simulink model "uut_vdif"  (R2012b)
settings: Solver=ode45  StartTime=0.0  StopTime=sim_time  RelTol=1e-3
libraries: xbsIndex_r4 x487, casper_library_delays x9, xps_library x1
(part 2 of 4)

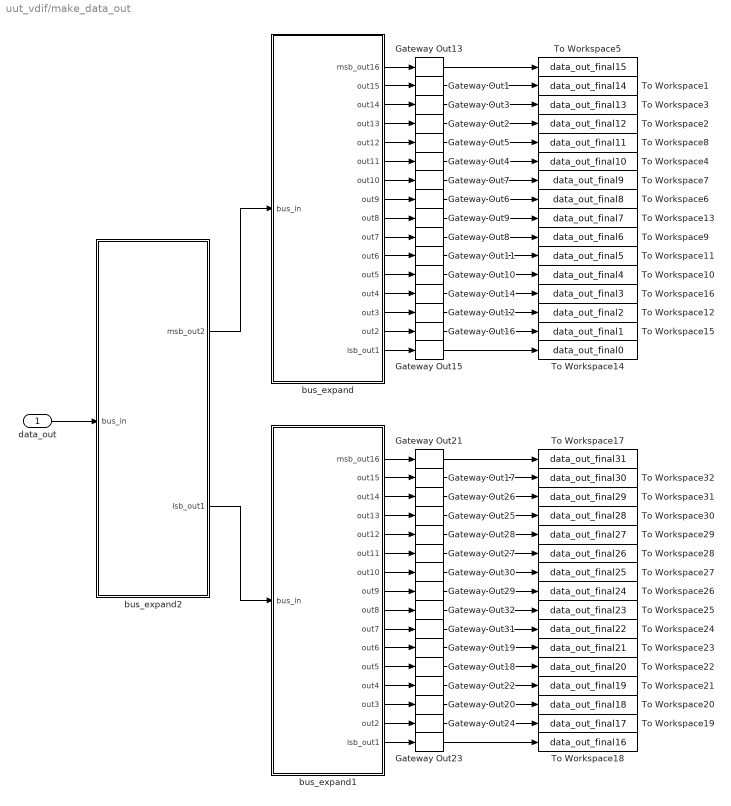
== system uut_vdif/make_data_out ==
  data_out : Inport
  Gateway Out{1..32} (32 alike) : xbsIndex_r4/Gateway Out  inherit_from_input=off  hdl_port=on  timing_constraint=None  locs_specified=off  LOCs={}  UseAsDAC=off  DACChannel='1'  block_type=gatewayout
  To Workspace1 : ToWorkspace  VariableName=data_out_final14  SampleTime=-1  SaveFormat=Timeseries
  To Workspace10 : ToWorkspace  VariableName=data_out_final4  SampleTime=-1  SaveFormat=Timeseries
  To Workspace11 : ToWorkspace  VariableName=data_out_final5  SampleTime=-1  SaveFormat=Timeseries
  To Workspace12 : ToWorkspace  VariableName=data_out_final2  SampleTime=-1  SaveFormat=Timeseries
  To Workspace13 : ToWorkspace  VariableName=data_out_final7  SampleTime=-1  SaveFormat=Timeseries
  To Workspace14 : ToWorkspace  VariableName=data_out_final0  SampleTime=-1  SaveFormat=Timeseries
  To Workspace15 : ToWorkspace  VariableName=data_out_final1  SampleTime=-1  SaveFormat=Timeseries
  To Workspace16 : ToWorkspace  VariableName=data_out_final3  SampleTime=-1  SaveFormat=Timeseries
  To Workspace17 : ToWorkspace  VariableName=data_out_final31  SampleTime=-1  SaveFormat=Timeseries
  To Workspace18 : ToWorkspace  VariableName=data_out_final16  SampleTime=-1  SaveFormat=Timeseries
  To Workspace19 : ToWorkspace  VariableName=data_out_final17  SampleTime=-1  SaveFormat=Timeseries
  To Workspace2 : ToWorkspace  VariableName=data_out_final12  SampleTime=-1  SaveFormat=Timeseries
  To Workspace20 : ToWorkspace  VariableName=data_out_final18  SampleTime=-1  SaveFormat=Timeseries
  To Workspace21 : ToWorkspace  VariableName=data_out_final19  SampleTime=-1  SaveFormat=Timeseries
  To Workspace22 : ToWorkspace  VariableName=data_out_final20  SampleTime=-1  SaveFormat=Timeseries
  To Workspace23 : ToWorkspace  VariableName=data_out_final21  SampleTime=-1  SaveFormat=Timeseries
  To Workspace24 : ToWorkspace  VariableName=data_out_final22  SampleTime=-1  SaveFormat=Timeseries
  To Workspace25 : ToWorkspace  VariableName=data_out_final23  SampleTime=-1  SaveFormat=Timeseries
  To Workspace26 : ToWorkspace  VariableName=data_out_final24  SampleTime=-1  SaveFormat=Timeseries
  To Workspace27 : ToWorkspace  VariableName=data_out_final25  SampleTime=-1  SaveFormat=Timeseries
  To Workspace28 : ToWorkspace  VariableName=data_out_final26  SampleTime=-1  SaveFormat=Timeseries
  To Workspace29 : ToWorkspace  VariableName=data_out_final27  SampleTime=-1  SaveFormat=Timeseries
  To Workspace3 : ToWorkspace  VariableName=data_out_final13  SampleTime=-1  SaveFormat=Timeseries
  To Workspace30 : ToWorkspace  VariableName=data_out_final28  SampleTime=-1  SaveFormat=Timeseries
  To Workspace31 : ToWorkspace  VariableName=data_out_final29  SampleTime=-1  SaveFormat=Timeseries
  To Workspace32 : ToWorkspace  VariableName=data_out_final30  SampleTime=-1  SaveFormat=Timeseries
  To Workspace4 : ToWorkspace  VariableName=data_out_final10  SampleTime=-1  SaveFormat=Timeseries
  To Workspace5 : ToWorkspace  VariableName=data_out_final15  SampleTime=-1  SaveFormat=Timeseries
  To Workspace6 : ToWorkspace  VariableName=data_out_final8  SampleTime=-1  SaveFormat=Timeseries
  To Workspace7 : ToWorkspace  VariableName=data_out_final9  SampleTime=-1  SaveFormat=Timeseries
  To Workspace8 : ToWorkspace  VariableName=data_out_final11  SampleTime=-1  SaveFormat=Timeseries
  To Workspace9 : ToWorkspace  VariableName=data_out_final6  SampleTime=-1  SaveFormat=Timeseries
  bus_expand : Subsystem  AncestorBlock=casper_library_flow_control/bus_expand  mask(bus_expand){mode=divisions of equal size, outputNum=16, outputWidth=2, outputBinaryPt=0, outputArithmeticType=0, show_format=off, outputToWorkspace=off, variablePrefix=out, outputToModelAsWell=on}
      mask prompts: outputNum "Number of outputs:"; outputWidth "Output width:"; outputBinaryPt "Output binary point position:"; outputArithmeticType "Output arithmetic type (ufix=0, fix=1, bool=2):"; show_format "Print format string?"; outputToWorkspace "Output to workspace?"; variablePrefix "Variable name prefix:"; outputToModelAsWell "Output to model as well?"
      mask help:
      | Expands a 'bus' made using a bus_create or Xilinx
      | concat block.
      | The input will be divided into the specified number
      | of outputs with the specified arithmetic types.
      | Divisions are made from most significant bit.
      mask init: same as uut_vdif/buffer_data/bus_expand
      settings: AttributesFormatString=16 outputs
      mask TypeOptions mode: divisions of equal size | divisions of arbitrary size
      mask Callback mode: bus_expand_callback();
      mask Callback outputWidth: bus_expand_callback();
      mask Callback outputToWorkspace: bus_expand_callback();
  bus_expand1 : Subsystem  AncestorBlock=casper_library_flow_control/bus_expand  mask(bus_expand){mode=divisions of equal size, outputNum=16, outputWidth=2, outputBinaryPt=0, outputArithmeticType=0, show_format=off, outputToWorkspace=off, variablePrefix=out, outputToModelAsWell=on}
      mask prompts: outputNum "Number of outputs:"; outputWidth "Output width:"; outputBinaryPt "Output binary point position:"; outputArithmeticType "Output arithmetic type (ufix=0, fix=1, bool=2):"; show_format "Print format string?"; outputToWorkspace "Output to workspace?"; variablePrefix "Variable name prefix:"; outputToModelAsWell "Output to model as well?"
      mask help:
      | Expands a 'bus' made using a bus_create or Xilinx
      | concat block.
      | The input will be divided into the specified number
      | of outputs with the specified arithmetic types.
      | Divisions are made from most significant bit.
      mask init: same as uut_vdif/buffer_data/bus_expand
      settings: AttributesFormatString=16 outputs
      mask TypeOptions mode: divisions of equal size | divisions of arbitrary size
      mask Callback mode: bus_expand_callback();
      mask Callback outputWidth: bus_expand_callback();
      mask Callback outputToWorkspace: bus_expand_callback();
  bus_expand2 : Subsystem  AncestorBlock=casper_library_flow_control/bus_expand  mask(bus_expand){mode=divisions of equal size, outputNum=2, outputWidth=32, outputBinaryPt=0, outputArithmeticType=0, show_format=off, outputToWorkspace=off, variablePrefix=out, outputToModelAsWell=on}
      mask prompts: outputNum "Number of outputs:"; outputWidth "Output width:"; outputBinaryPt "Output binary point position:"; outputArithmeticType "Output arithmetic type (ufix=0, fix=1, bool=2):"; show_format "Print format string?"; outputToWorkspace "Output to workspace?"; variablePrefix "Variable name prefix:"; outputToModelAsWell "Output to model as well?"
      mask help:
      | Expands a 'bus' made using a bus_create or Xilinx
      | concat block.
      | The input will be divided into the specified number
      | of outputs with the specified arithmetic types.
      | Divisions are made from most significant bit.
      mask init: same as uut_vdif/buffer_data/bus_expand
      settings: AttributesFormatString=2 outputs
      mask TypeOptions mode: divisions of equal size | divisions of arbitrary size
      mask Callback mode: bus_expand_callback();
      mask Callback outputWidth: bus_expand_callback();
      mask Callback outputToWorkspace: bus_expand_callback();
  wires:
  Gateway Out13/1 -> To Workspace5/1
  bus_expand/1(msb_out16) -> Gateway Out13/1
  bus_expand/2(out15) -> Gateway Out1/1
  Gateway Out1/1 -> To Workspace1/1
  Gateway Out3/1 -> To Workspace3/1
  bus_expand/3(out14) -> Gateway Out3/1
  bus_expand/4(out13) -> Gateway Out2/1
  Gateway Out2/1 -> To Workspace2/1
  Gateway Out5/1 -> To Workspace8/1
  bus_expand/5(out12) -> Gateway Out5/1
  bus_expand/6(out11) -> Gateway Out4/1
  Gateway Out4/1 -> To Workspace4/1
  Gateway Out7/1 -> To Workspace7/1
  bus_expand/7(out10) -> Gateway Out7/1
  bus_expand/8(out9) -> Gateway Out6/1
  Gateway Out6/1 -> To Workspace6/1
  Gateway Out9/1 -> To Workspace13/1
  bus_expand/9(out8) -> Gateway Out9/1
  bus_expand/10(out7) -> Gateway Out8/1
  Gateway Out8/1 -> To Workspace9/1
  Gateway Out11/1 -> To Workspace11/1
  bus_expand/11(out6) -> Gateway Out11/1
  bus_expand/12(out5) -> Gateway Out10/1
  Gateway Out10/1 -> To Workspace10/1
  Gateway Out14/1 -> To Workspace16/1
  bus_expand/13(out4) -> Gateway Out14/1
  bus_expand/14(out3) -> Gateway Out12/1
  Gateway Out12/1 -> To Workspace12/1
  Gateway Out16/1 -> To Workspace15/1
  bus_expand/15(out2) -> Gateway Out16/1
  bus_expand/16(lsb_out1) -> Gateway Out15/1
  Gateway Out15/1 -> To Workspace14/1
  bus_expand1/1(msb_out16) -> Gateway Out21/1
  bus_expand1/2(out15) -> Gateway Out17/1
  bus_expand1/3(out14) -> Gateway Out26/1
  bus_expand1/4(out13) -> Gateway Out25/1
  bus_expand1/5(out12) -> Gateway Out28/1
  bus_expand1/6(out11) -> Gateway Out27/1
  bus_expand1/7(out10) -> Gateway Out30/1
  bus_expand1/8(out9) -> Gateway Out29/1
  bus_expand1/9(out8) -> Gateway Out32/1
  bus_expand1/10(out7) -> Gateway Out31/1
  bus_expand1/11(out6) -> Gateway Out19/1
  bus_expand1/12(out5) -> Gateway Out18/1
  bus_expand1/13(out4) -> Gateway Out22/1
  bus_expand1/14(out3) -> Gateway Out20/1
  bus_expand1/15(out2) -> Gateway Out24/1
  bus_expand1/16(lsb_out1) -> Gateway Out23/1
  data_out/1 -> bus_expand2/1(bus_in)
  bus_expand2/1(msb_out2) -> bus_expand/1(bus_in)
  bus_expand2/2(lsb_out1) -> bus_expand1/1(bus_in)
  Gateway Out21/1 -> To Workspace17/1
  Gateway Out17/1 -> To Workspace32/1
  Gateway Out26/1 -> To Workspace31/1
  Gateway Out25/1 -> To Workspace30/1
  Gateway Out28/1 -> To Workspace29/1
  Gateway Out27/1 -> To Workspace28/1
  Gateway Out30/1 -> To Workspace27/1
  Gateway Out29/1 -> To Workspace26/1
  Gateway Out32/1 -> To Workspace25/1
  Gateway Out31/1 -> To Workspace24/1
  Gateway Out19/1 -> To Workspace23/1
  Gateway Out18/1 -> To Workspace22/1
  Gateway Out22/1 -> To Workspace21/1
  Gateway Out20/1 -> To Workspace20/1
  Gateway Out24/1 -> To Workspace19/1
  Gateway Out23/1 -> To Workspace18/1

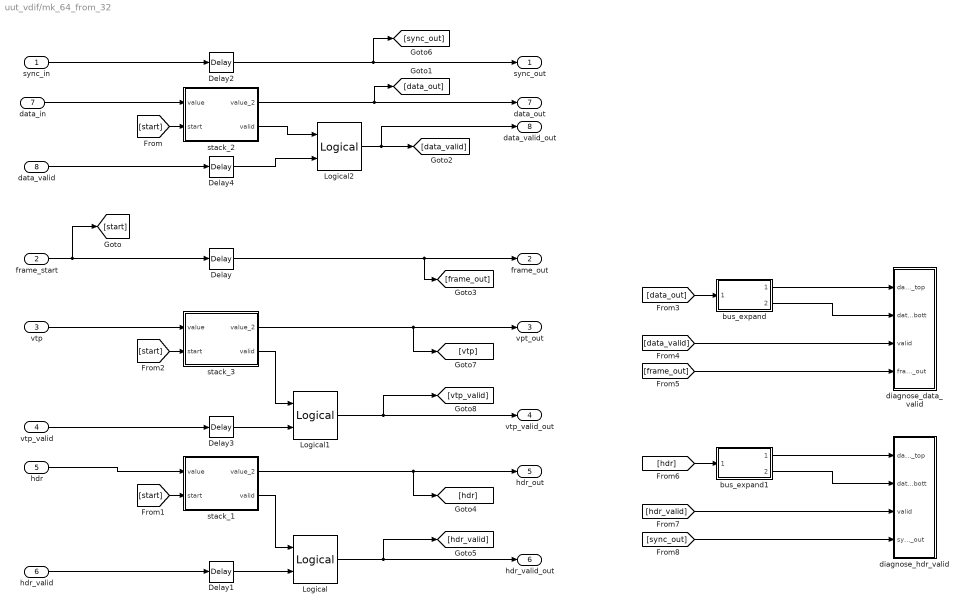
== system uut_vdif/mk_64_from_32 ==
  sync_in : Inport
  frame_start : Inport  Port=2
  vtp : Inport  Port=3
  vtp_valid : Inport  Port=4
  hdr : Inport  Port=5
  hdr_valid : Inport  Port=6
  data_in : Inport  Port=7
  data_valid : Inport  Port=8
  Delay{,1..4} (5 alike) : xbsIndex_r4/Delay  rst=off  infoeditControl=Selection of Reset will increase slice count due to use of real FFs and instead of SRLs  en=off  latency=2  dbl_ovrd=off  reg_retiming=off  block_type=delay
  Logical : xbsIndex_r4/Logical  logical_function=AND  inputs=2  en=off  latency=0  precision=Full  arith_type=Unsigned  n_bits=16  bin_pt=0  align_bp=on  dbl_ovrd=off  block_type=logical
  Logical1 : xbsIndex_r4/Logical  logical_function=AND  inputs=2  en=off  latency=0  precision=Full  arith_type=Unsigned  n_bits=16  bin_pt=0  align_bp=on  dbl_ovrd=off  block_type=logical
  Logical2 : xbsIndex_r4/Logical  logical_function=AND  inputs=2  en=off  latency=0  precision=Full  arith_type=Unsigned  n_bits=16  bin_pt=0  align_bp=on  dbl_ovrd=off  block_type=logical
  bus_expand : Subsystem  AncestorBlock=casper_library_flow_control/bus_expand  mask(bus_expand){mode=divisions of equal size, outputNum=2, outputWidth=32, outputBinaryPt=0, outputArithmeticType=0, show_format=off, outputToWorkspace=off, variablePrefix=out, outputToModelAsWell=on}
      mask prompts: outputNum "Number of outputs:"; outputWidth "Output width:"; outputBinaryPt "Output binary point position:"; outputArithmeticType "Output arithmetic type (ufix=0, fix=1, bool=2):"; show_format "Print format string?"; outputToWorkspace "Output to workspace?"; variablePrefix "Variable name prefix:"; outputToModelAsWell "Output to model as well?"
      mask help:
      | Expands a 'bus' made using a bus_create or Xilinx
      | concat block.
      | The input will be divided into the specified number
      | of outputs with the specified arithmetic types.
      | Divisions are made from most significant bit.
      mask init: same as uut_vdif/buffer_data/bus_expand
      settings: AttributesFormatString=2 outputs
      mask TypeOptions mode: divisions of equal size | divisions of arbitrary size
      mask Callback mode: bus_expand_callback();
      mask Callback outputWidth: bus_expand_callback();
      mask Callback outputToWorkspace: bus_expand_callback();
  bus_expand1 : Subsystem  AncestorBlock=casper_library_flow_control/bus_expand  mask(bus_expand){mode=divisions of equal size, outputNum=2, outputWidth=32, outputBinaryPt=0, outputArithmeticType=0, show_format=off, outputToWorkspace=off, variablePrefix=out, outputToModelAsWell=on}
      mask prompts: outputNum "Number of outputs:"; outputWidth "Output width:"; outputBinaryPt "Output binary point position:"; outputArithmeticType "Output arithmetic type (ufix=0, fix=1, bool=2):"; show_format "Print format string?"; outputToWorkspace "Output to workspace?"; variablePrefix "Variable name prefix:"; outputToModelAsWell "Output to model as well?"
      mask help:
      | Expands a 'bus' made using a bus_create or Xilinx
      | concat block.
      | The input will be divided into the specified number
      | of outputs with the specified arithmetic types.
      | Divisions are made from most significant bit.
      mask init: same as uut_vdif/buffer_data/bus_expand
      settings: AttributesFormatString=2 outputs
      mask TypeOptions mode: divisions of equal size | divisions of arbitrary size
      mask Callback mode: bus_expand_callback();
      mask Callback outputWidth: bus_expand_callback();
      mask Callback outputToWorkspace: bus_expand_callback();
  diagnose_data_valid : Subsystem
  diagnose_hdr_valid : Subsystem
  stack_1 : Subsystem
      mask help: stacks 2 samples together, based on a flag that indicates the start or the first sample of data to be stacked. outputs the stacked data and a valid signal, such that on any given valid signal the data represents the newest data in the top half and the oldest data in the lower half. Therefore given a data stream starting with 0, increasing by 1 every clock cycle I would expect the first data valid to indicate a piece of data with the value 0 in the low bits, 1 in the high, and the next sample having 2 in the low bits 3 in the high, etc.
  stack_2 : Subsystem
      mask help: stacks 2 samples together, based on a flag that indicates the start or the first sample of data to be stacked. outputs the stacked data and a valid signal, such that on any given valid signal the data represents the newest data in the top half and the oldest data in the lower half. Therefore given a data stream starting with 0, increasing by 1 every clock cycle I would expect the first data valid to indicate a piece of data with the value 0 in the low bits, 1 in the high, and the next sample having 2 in the low bits 3 in the high, etc.
  stack_3 : Subsystem
      mask help: stacks 2 samples together, based on a flag that indicates the start or the first sample of data to be stacked. outputs the stacked data and a valid signal, such that on any given valid signal the data represents the newest data in the top half and the oldest data in the lower half. Therefore given a data stream starting with 0, increasing by 1 every clock cycle I would expect the first data valid to indicate a piece of data with the value 0 in the low bits, 1 in the high, and the next sample having 2 in the low bits 3 in the high, etc.
  sync_out : Outport
  frame_out : Outport  Port=2
  vpt_out : Outport  Port=3
  vtp_valid_out : Outport  Port=4
  hdr_out : Outport  Port=5
  hdr_valid_out : Outport  Port=6
  data_out : Outport  Port=7
  data_valid_out : Outport  Port=8
  wires:
  data_in/1 -> stack_2/1(value)
  frame_start/1 -> [start], Delay/1
  [start] -> stack_2/2(start)
  sync_in/1 -> Delay2/1
  stack_2/1(value_2) -> data_out/1, [data_out]
  [start] -> stack_1/2(start)
  stack_1/1(value_2) -> hdr_out/1, [hdr]
  stack_1/2(valid) -> Logical/1
  Delay/1 -> [frame_out], frame_out/1
  bus_expand/2(lsb_out1) -> diagnose_data_valid/2(data_bott)
  bus_expand/1(msb_out2) -> diagnose_data_valid/1(data_top)
  [data_valid] -> diagnose_data_valid/3(valid)
  [frame_out] -> diagnose_data_valid/4(frame_start_out)
  [data_out] -> bus_expand/1(bus_in)
  bus_expand1/2(lsb_out1) -> diagnose_hdr_valid/2(data_bott)
  bus_expand1/1(msb_out2) -> diagnose_hdr_valid/1(data_top)
  [hdr_valid] -> diagnose_hdr_valid/3(valid)
  [sync_out] -> diagnose_hdr_valid/4(sync_out)
  [hdr] -> bus_expand1/1(bus_in)
  Logical/1 -> hdr_valid_out/1, [hdr_valid]
  Delay1/1 -> Logical/2
  Delay2/1 -> [sync_out], sync_out/1
  [start] -> stack_3/2(start)
  stack_3/1(value_2) -> vpt_out/1, [vtp]
  stack_3/2(valid) -> Logical1/1
  Logical1/1 -> vtp_valid_out/1, [vtp_valid]
  Delay3/1 -> Logical1/2
  vtp/1 -> stack_3/1(value)
  vtp_valid/1 -> Delay3/1
  hdr/1 -> stack_1/1(value)
  hdr_valid/1 -> Delay1/1
  data_valid/1 -> Delay4/1
  Delay4/1 -> Logical2/2
  stack_2/2(valid) -> Logical2/1
  Logical2/1 -> data_valid_out/1, [data_valid]

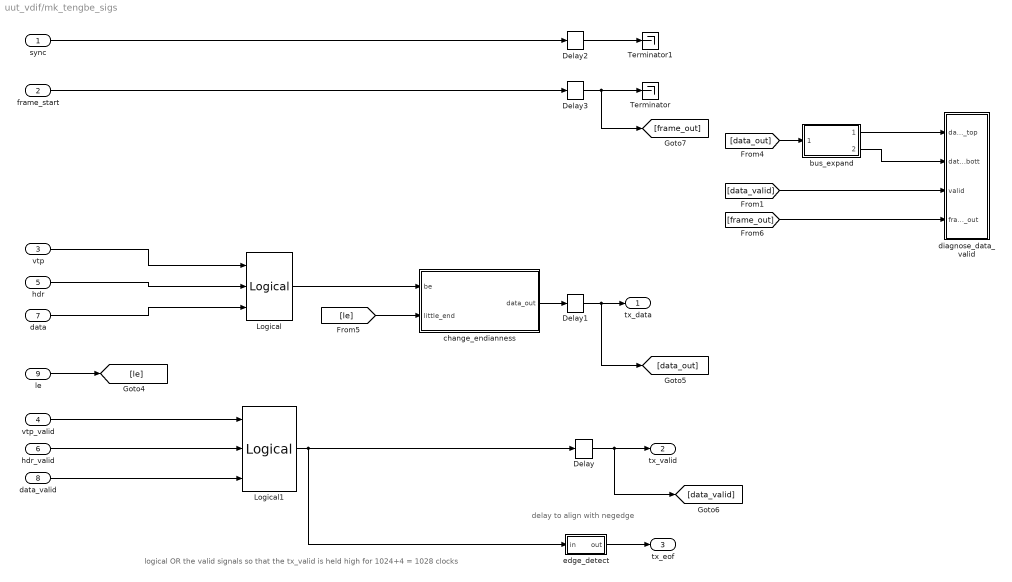
== system uut_vdif/mk_tengbe_sigs ==
  note: logical OR the valid signals so that the
      | tx_valid is held high for 1024+4 = 1028 clocks
  note: delay to align with
      | negedge
  sync : Inport
  frame_start : Inport  Port=2
  vtp : Inport  Port=3
  vtp_valid : Inport  Port=4
  hdr : Inport  Port=5
  hdr_valid : Inport  Port=6
  data : Inport  Port=7
  data_valid : Inport  Port=8
  le : Inport  Port=9
  Delay{,1..3} (4 alike) : xbsIndex_r4/Delay  rst=off  infoeditControl=Selection of Reset will increase slice count due to use of real FFs and instead of SRLs  en=off  latency=1  dbl_ovrd=off  reg_retiming=off  block_type=delay
  Logical : xbsIndex_r4/Logical  logical_function=XOR  inputs=3  en=off  latency=0  precision=Full  arith_type=Unsigned  n_bits=16  bin_pt=0  align_bp=on  dbl_ovrd=off  block_type=logical
  Logical1 : xbsIndex_r4/Logical  logical_function=XOR  inputs=3  en=off  latency=0  precision=Full  arith_type=Unsigned  n_bits=16  bin_pt=0  align_bp=on  dbl_ovrd=off  block_type=logical
  Terminator : Terminator
  Terminator1 : Terminator
  bus_expand : Subsystem  AncestorBlock=casper_library_flow_control/bus_expand  mask(bus_expand){mode=divisions of equal size, outputNum=2, outputWidth=32, outputBinaryPt=0, outputArithmeticType=0, show_format=off, outputToWorkspace=off, variablePrefix=out, outputToModelAsWell=on}
      mask prompts: outputNum "Number of outputs:"; outputWidth "Output width:"; outputBinaryPt "Output binary point position:"; outputArithmeticType "Output arithmetic type (ufix=0, fix=1, bool=2):"; show_format "Print format string?"; outputToWorkspace "Output to workspace?"; variablePrefix "Variable name prefix:"; outputToModelAsWell "Output to model as well?"
      mask help:
      | Expands a 'bus' made using a bus_create or Xilinx
      | concat block.
      | The input will be divided into the specified number
      | of outputs with the specified arithmetic types.
      | Divisions are made from most significant bit.
      mask init: same as uut_vdif/buffer_data/bus_expand
      settings: AttributesFormatString=2 outputs
      mask TypeOptions mode: divisions of equal size | divisions of arbitrary size
      mask Callback mode: bus_expand_callback();
      mask Callback outputWidth: bus_expand_callback();
      mask Callback outputToWorkspace: bus_expand_callback();
  change_endianness : Subsystem
  diagnose_data_valid : Subsystem
  edge_detect : Subsystem  AncestorBlock=casper_library_misc/edge_detect  mask(edge_detect){edge=Falling, polarity=Active High, x_in=[0 0.08 0.08 0.16 0.16 0.24 0.24 0.32 0.32 0.4], y_in=[-1 -1  1  1  1  1  1  1  1  1], x_out=[0.6 0.68 0.68 0.76 0.76 0.84 0.84 0.92 0.92 1], y_out=[-1 -1  1  1 -1 -1 -1 -1 -1 -1]}
      mask prompts: edge "Edge Type"; polarity "Output Polarity"; x_in "Input X Positions"; y_in "Input Y Positions"; x_out "Output X Positions"; y_out "Output Y Positions"
      mask help: Output is active for one-cycle after each edge of the specified type (i.e. rising, falling or both).
      mask init:
      | edge_detect_init(gcb,...
      |     'edge',edge,...
      |     'polarity',polarity,...
      |     'x_in',x_in,...
      |     'x_out',x_out,...
      |     'y_in',y_in,...
      |     'y_out',y_out);
      | 
      | x_in_num=str2num(getfield(getfield(get_param(gcb,'UserData'),'parameters'),'x_in'));
      | x_out_num=str2num(getfield(getfield(get_param(gcb,'UserData'),'parameters'),'x_out'));
      | y_in_num=str2num(getfield(getfield(get_param(gcb,'UserData'),'parameters'),'y_in'));
      | y_out_num=str2num(getfield(getfield(get_param(gcb,'UserData'),'parameters'),'y_out'));
      settings: AttributesFormatString=|
      | falling edges
      | active high
      mask Help: Output is active for one-cycle after each edge of the specified type (i.e. rising, falling, or both).  Latency is zero.
      mask TypeOptions edge: Rising | Falling | Both
      mask TypeOptions polarity: Active High | Active Low
      mask Display:
      | plot(x_in_num,0.5+y_in_num*0.2);
      | plot(x_out_num,0.5+y_out_num*0.2);
  tx_data : Outport
  tx_valid : Outport  Port=2
  tx_eof : Outport  Port=3
  wires:
  edge_detect/1(out) -> tx_eof/1
  Logical1/1 -> edge_detect/1(in), Delay/1
  Delay/1 -> [data_valid], tx_valid/1
  Logical/1 -> change_endianness/1(be)
  change_endianness/1(data_out) -> Delay1/1
  [le] -> change_endianness/2(little_end)
  Delay2/1 -> Terminator1/1
  sync/1 -> Delay2/1
  Delay1/1 -> [data_out], tx_data/1
  frame_start/1 -> Delay3/1
  Delay3/1 -> [frame_out], Terminator/1
  bus_expand/2(lsb_out1) -> diagnose_data_valid/2(data_bott)
  bus_expand/1(msb_out2) -> diagnose_data_valid/1(data_top)
  [data_valid] -> diagnose_data_valid/3(valid)
  [frame_out] -> diagnose_data_valid/4(frame_start_out)
  [data_out] -> bus_expand/1(bus_in)
  hdr/1 -> Logical/2
  vtp/1 -> Logical/1
  data/1 -> Logical/3
  le/1 -> [le]
  vtp_valid/1 -> Logical1/1
  hdr_valid/1 -> Logical1/2
  data_valid/1 -> Logical1/3

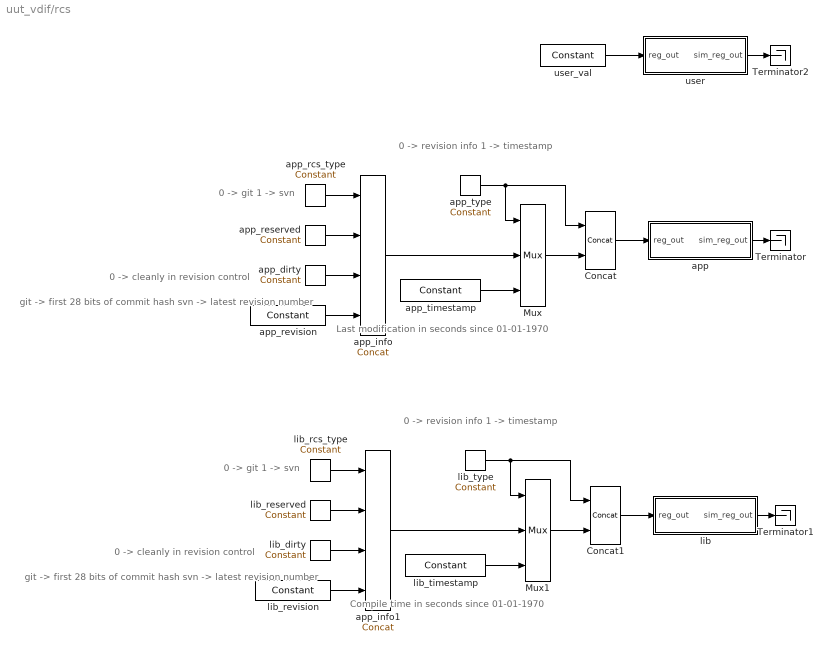
== system uut_vdif/rcs ==
  note: 0 -> revision info
      | 1 -> timestamp
  note: Last modification
      | in seconds since
      | 01-01-1970
  note: 0 -> git
      | 1 -> svn
  note: 0 -> cleanly in revision control
  note: git -> first 28 bits of commit hash
      | svn -> latest revision number
  note: 0 -> revision info
      | 1 -> timestamp
  note: Compile time
      | in seconds since
      | 01-01-1970
  note: 0 -> git
      | 1 -> svn
  note: 0 -> cleanly in revision control
  note: git -> first 28 bits of commit hash
      | svn -> latest revision number
  Concat : xbsIndex_r4/Concat  num_inputs=2  dbl_ovrd=off  block_type=concat
  Concat1 : xbsIndex_r4/Concat  num_inputs=2  dbl_ovrd=off  block_type=concat
  Mux : xbsIndex_r4/Mux  inputs=2  en=off  latency=0  precision=Full  arith_type=Unsigned  n_bits=16  bin_pt=14  quantization=Truncate  overflow=Wrap  dbl_ovrd=off  block_type=mux
      settings: block_version=11.4
  Mux1 : xbsIndex_r4/Mux  inputs=2  en=off  latency=0  precision=Full  arith_type=Unsigned  n_bits=16  bin_pt=14  quantization=Truncate  overflow=Wrap  dbl_ovrd=off  block_type=mux
      settings: block_version=11.4
  Terminator : Terminator
  Terminator1 : Terminator
  Terminator2 : Terminator
  app : Subsystem  Tag=xps:sw_reg  mask{io_dir=To Processor, arith_type=Unsigned, bitwidth=32, bin_pt=0, sample_period=1, latency=0}
      mask prompts: io_dir "I/O direction"; arith_type "Data Type"; bitwidth "Data bitwidth"; bin_pt "Data binary point"; sample_period "Sample period"
      mask init:
      | gw_name = clear_name(gcb);
      | config.source = str2func('software_register_init');
      | config.toplevel = gcb;
      | xBlock( config, {io_dir, arith_type, bitwidth, bin_pt, ... 
      |     sample_period, gw_name, latency});
      mask TypeOptions io_dir: From Processor | To Processor
      mask TypeOptions arith_type: Unsigned | Signed  (2's comp)
  app_dirty : xbsIndex_r4/Constant  const=1  gui_display_data_type=Fixed-point  arith_type=Unsigned  n_bits=1  bin_pt=0  preci_type=Single  exp_width=8  frac_width=24  explicit_period=on  period=1  equ=P=C  opselect=C  inp2=PCIN>>17  opr=+  inp1=P  carry=CIN  dbl_ovrd=off  block_type=constant
      settings: block_version=11.4
  app_info : xbsIndex_r4/Concat  num_inputs=4  dbl_ovrd=off  block_type=concat
  app_info1 : xbsIndex_r4/Concat  num_inputs=4  dbl_ovrd=off  block_type=concat
  app_rcs_type : xbsIndex_r4/Constant  const=0  gui_display_data_type=Fixed-point  arith_type=Unsigned  n_bits=1  bin_pt=0  preci_type=Single  exp_width=8  frac_width=24  explicit_period=on  period=1  equ=P=C  opselect=C  inp2=PCIN>>17  opr=+  inp1=P  carry=CIN  dbl_ovrd=off  block_type=constant
      settings: block_version=11.4
  app_reserved : xbsIndex_r4/Constant  const=0  gui_display_data_type=Fixed-point  arith_type=Unsigned  n_bits=1  bin_pt=0  preci_type=Single  exp_width=8  frac_width=24  explicit_period=on  period=1  equ=P=C  opselect=C  inp2=PCIN>>17  opr=+  inp1=P  carry=CIN  dbl_ovrd=off  block_type=constant
      settings: block_version=11.4
  app_revision : xbsIndex_r4/Constant  const=0  gui_display_data_type=Fixed-point  arith_type=Unsigned  n_bits=28  bin_pt=0  preci_type=Single  exp_width=8  frac_width=24  explicit_period=on  period=1  equ=P=C  opselect=C  inp2=PCIN>>17  opr=+  inp1=P  carry=CIN  dbl_ovrd=off  block_type=constant
      settings: block_version=11.4
  app_timestamp : xbsIndex_r4/Constant  const=1440776925  gui_display_data_type=Fixed-point  arith_type=Unsigned  n_bits=31  bin_pt=0  preci_type=Single  exp_width=8  frac_width=24  explicit_period=on  period=1  equ=P=C  opselect=C  inp2=PCIN>>17  opr=+  inp1=P  carry=CIN  dbl_ovrd=off  block_type=constant
      settings: block_version=11.4
  app_type : xbsIndex_r4/Constant  const=1  gui_display_data_type=Fixed-point  arith_type=Unsigned  n_bits=1  bin_pt=0  preci_type=Single  exp_width=8  frac_width=24  explicit_period=on  period=1  equ=P=C  opselect=C  inp2=PCIN>>17  opr=+  inp1=P  carry=CIN  dbl_ovrd=off  block_type=constant
      settings: block_version=11.4
  lib : Subsystem  Tag=xps:sw_reg  mask{io_dir=To Processor, arith_type=Unsigned, bitwidth=32, bin_pt=0, sample_period=1, latency=0}
      mask prompts: io_dir "I/O direction"; arith_type "Data Type"; bitwidth "Data bitwidth"; bin_pt "Data binary point"; sample_period "Sample period"
      mask init:
      | gw_name = clear_name(gcb);
      | config.source = str2func('software_register_init');
      | config.toplevel = gcb;
      | xBlock( config, {io_dir, arith_type, bitwidth, bin_pt, ... 
      |     sample_period, gw_name, latency});
      mask TypeOptions io_dir: From Processor | To Processor
      mask TypeOptions arith_type: Unsigned | Signed  (2's comp)
  lib_dirty : xbsIndex_r4/Constant  const=1  gui_display_data_type=Fixed-point  arith_type=Unsigned  n_bits=1  bin_pt=0  preci_type=Single  exp_width=8  frac_width=24  explicit_period=on  period=1  equ=P=C  opselect=C  inp2=PCIN>>17  opr=+  inp1=P  carry=CIN  dbl_ovrd=off  block_type=constant
      settings: block_version=11.4
  lib_rcs_type : xbsIndex_r4/Constant  const=0  gui_display_data_type=Fixed-point  arith_type=Unsigned  n_bits=1  bin_pt=0  preci_type=Single  exp_width=8  frac_width=24  explicit_period=on  period=1  equ=P=C  opselect=C  inp2=PCIN>>17  opr=+  inp1=P  carry=CIN  dbl_ovrd=off  block_type=constant
      settings: block_version=11.4
  lib_reserved : xbsIndex_r4/Constant  const=0  gui_display_data_type=Fixed-point  arith_type=Unsigned  n_bits=1  bin_pt=0  preci_type=Single  exp_width=8  frac_width=24  explicit_period=on  period=1  equ=P=C  opselect=C  inp2=PCIN>>17  opr=+  inp1=P  carry=CIN  dbl_ovrd=off  block_type=constant
      settings: block_version=11.4
  lib_revision : xbsIndex_r4/Constant  const=hex2dec('a288ff3')  gui_display_data_type=Fixed-point  arith_type=Unsigned  n_bits=28  bin_pt=0  preci_type=Single  exp_width=8  frac_width=24  explicit_period=on  period=1  equ=P=C  opselect=C  inp2=PCIN>>17  opr=+  inp1=P  carry=CIN  dbl_ovrd=off  block_type=constant
      settings: block_version=11.4
  lib_timestamp : xbsIndex_r4/Constant  const=1440763282  gui_display_data_type=Fixed-point  arith_type=Unsigned  n_bits=31  bin_pt=0  preci_type=Single  exp_width=8  frac_width=24  explicit_period=on  period=1  equ=P=C  opselect=C  inp2=PCIN>>17  opr=+  inp1=P  carry=CIN  dbl_ovrd=off  block_type=constant
      settings: block_version=11.4
  lib_type : xbsIndex_r4/Constant  const=0  gui_display_data_type=Fixed-point  arith_type=Unsigned  n_bits=1  bin_pt=0  preci_type=Single  exp_width=8  frac_width=24  explicit_period=on  period=1  equ=P=C  opselect=C  inp2=PCIN>>17  opr=+  inp1=P  carry=CIN  dbl_ovrd=off  block_type=constant
      settings: block_version=11.4
  user : Subsystem  Tag=xps:sw_reg  mask{io_dir=To Processor, arith_type=Unsigned, bitwidth=32, bin_pt=0, sample_period=1, latency=0}
      mask prompts: io_dir "I/O direction"; arith_type "Data Type"; bitwidth "Data bitwidth"; bin_pt "Data binary point"; sample_period "Sample period"
      mask init:
      | gw_name = clear_name(gcb);
      | config.source = str2func('software_register_init');
      | config.toplevel = gcb;
      | xBlock( config, {io_dir, arith_type, bitwidth, bin_pt, ... 
      |     sample_period, gw_name, latency});
      mask TypeOptions io_dir: From Processor | To Processor
      mask TypeOptions arith_type: Unsigned | Signed  (2's comp)
  user_val : xbsIndex_r4/Constant  const=user_val  gui_display_data_type=Fixed-point  arith_type=Unsigned  n_bits=32  bin_pt=0  preci_type=Single  exp_width=8  frac_width=24  explicit_period=off  period=1  equ=P=C  opselect=C  inp2=PCIN>>17  opr=+  inp1=P  carry=CIN  dbl_ovrd=off  block_type=constant
      settings: block_version=11.4
  wires:
  app/1(sim_reg_out) -> Terminator/1
  user/1(sim_reg_out) -> Terminator2/1
  user_val/1 -> user/1(reg_out)
  app_rcs_type/1 -> app_info/1
  app_reserved/1 -> app_info/2
  app_dirty/1 -> app_info/3
  app_revision/1 -> app_info/4
  app_type/1 -> Concat/1, Mux/1
  app_info/1 -> Mux/2
  app_timestamp/1 -> Mux/3
  Mux/1 -> Concat/2
  Concat/1 -> app/1(reg_out)
  lib/1(sim_reg_out) -> Terminator1/1
  lib_rcs_type/1 -> app_info1/1
  lib_reserved/1 -> app_info1/2
  lib_dirty/1 -> app_info1/3
  lib_revision/1 -> app_info1/4
  lib_type/1 -> Concat1/1, Mux1/1
  app_info1/1 -> Mux1/2
  lib_timestamp/1 -> Mux1/3
  Mux1/1 -> Concat1/2
  Concat1/1 -> lib/1(reg_out)

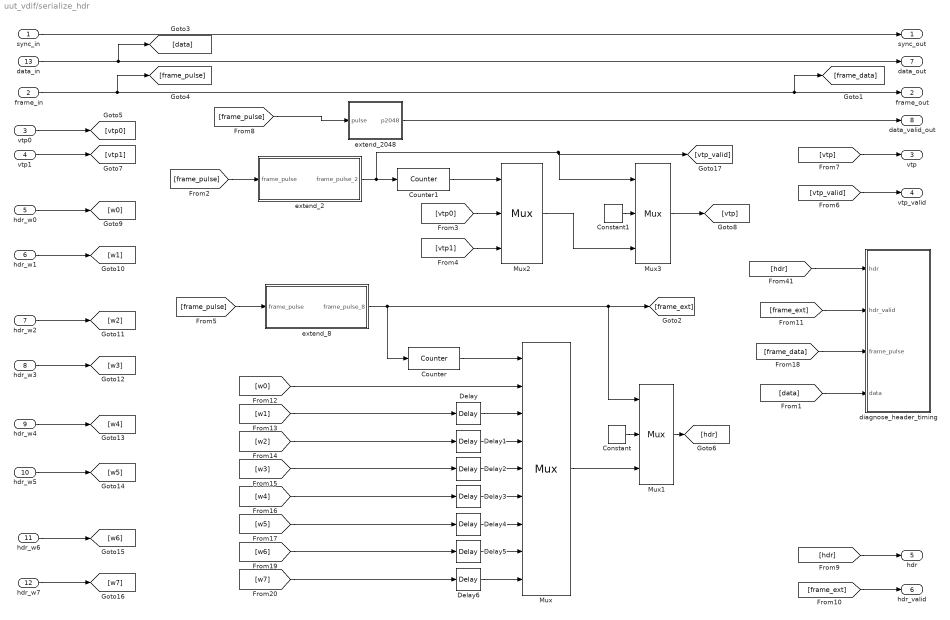
== system uut_vdif/serialize_hdr ==
  sync_in : Inport
  frame_in : Inport  Port=2
  vtp0 : Inport  Port=3
  vtp1 : Inport  Port=4
  " hdr_w0" : Inport  Port=5
  " hdr_w1" : Inport  Port=6
  " hdr_w2" : Inport  Port=7
  " hdr_w3" : Inport  Port=8
  " hdr_w4" : Inport  Port=9
  " hdr_w5" : Inport  Port=10
  " hdr_w6" : Inport  Port=11
  " hdr_w7" : Inport  Port=12
  " data_in" : Inport  Port=13
  Constant : xbsIndex_r4/Constant  const=0  gui_display_data_type=Fixed-point  arith_type=Unsigned  n_bits=32  bin_pt=0  preci_type=Single  exp_width=8  frac_width=24  explicit_period=on  period=1  equ=P=C  opselect=C  inp2=PCIN>>17  opr=+  inp1=P  carry=CIN  dbl_ovrd=off  block_type=constant
  Constant1 : xbsIndex_r4/Constant  const=0  gui_display_data_type=Fixed-point  arith_type=Unsigned  n_bits=32  bin_pt=0  preci_type=Single  exp_width=8  frac_width=24  explicit_period=on  period=1  equ=P=C  opselect=C  inp2=PCIN>>17  opr=+  inp1=P  carry=CIN  dbl_ovrd=off  block_type=constant
  Counter : xbsIndex_r4/Counter  cnt_type=Free Running  cnt_to=Inf  operation=Up  start_count=0  cnt_by_val=1  arith_type=Unsigned  n_bits=3  bin_pt=0  load_pin=off  rst=off  en=on  explicit_period=on  period=1  dbl_ovrd=off  use_behavioral_HDL=off  implementation=Fabric  block_type=counter
  Counter1 : xbsIndex_r4/Counter  cnt_type=Free Running  cnt_to=Inf  operation=Up  start_count=0  cnt_by_val=1  arith_type=Unsigned  n_bits=1  bin_pt=0  load_pin=off  rst=off  en=on  explicit_period=on  period=1  dbl_ovrd=off  use_behavioral_HDL=off  implementation=Fabric  block_type=counter
  Delay : xbsIndex_r4/Delay  rst=off  infoeditControl=Selection of Reset will increase slice count due to use of real FFs and instead of SRLs  en=off  latency=1  dbl_ovrd=off  reg_retiming=off  block_type=delay
  Delay1 : xbsIndex_r4/Delay  rst=off  infoeditControl=Selection of Reset will increase slice count due to use of real FFs and instead of SRLs  en=off  latency=2  dbl_ovrd=off  reg_retiming=off  block_type=delay
  Delay2 : xbsIndex_r4/Delay  rst=off  infoeditControl=Selection of Reset will increase slice count due to use of real FFs and instead of SRLs  en=off  latency=3  dbl_ovrd=off  reg_retiming=off  block_type=delay
  Delay3 : xbsIndex_r4/Delay  rst=off  infoeditControl=Selection of Reset will increase slice count due to use of real FFs and instead of SRLs  en=off  latency=4  dbl_ovrd=off  reg_retiming=off  block_type=delay
  Delay4 : xbsIndex_r4/Delay  rst=off  infoeditControl=Selection of Reset will increase slice count due to use of real FFs and instead of SRLs  en=off  latency=5  dbl_ovrd=off  reg_retiming=off  block_type=delay
  Delay5 : xbsIndex_r4/Delay  rst=off  infoeditControl=Selection of Reset will increase slice count due to use of real FFs and instead of SRLs  en=off  latency=6  dbl_ovrd=off  reg_retiming=off  block_type=delay
  Delay6 : xbsIndex_r4/Delay  rst=off  infoeditControl=Selection of Reset will increase slice count due to use of real FFs and instead of SRLs  en=off  latency=7  dbl_ovrd=off  reg_retiming=off  block_type=delay
  Mux : xbsIndex_r4/Mux  inputs=8  en=off  latency=0  precision=Full  arith_type=Unsigned  n_bits=16  bin_pt=14  quantization=Truncate  overflow=Wrap  dbl_ovrd=off  block_type=mux
  Mux1 : xbsIndex_r4/Mux  inputs=2  en=off  latency=0  precision=Full  arith_type=Unsigned  n_bits=16  bin_pt=14  quantization=Truncate  overflow=Wrap  dbl_ovrd=off  block_type=mux
  Mux2 : xbsIndex_r4/Mux  inputs=2  en=off  latency=0  precision=Full  arith_type=Unsigned  n_bits=16  bin_pt=14  quantization=Truncate  overflow=Wrap  dbl_ovrd=off  block_type=mux
  Mux3 : xbsIndex_r4/Mux  inputs=2  en=off  latency=0  precision=Full  arith_type=Unsigned  n_bits=16  bin_pt=14  quantization=Truncate  overflow=Wrap  dbl_ovrd=off  block_type=mux
  diagnose_header_timing : Subsystem
  extend_2 : Subsystem
  extend_2048 : Subsystem
  extend_8 : Subsystem
  sync_out : Outport
  frame_out : Outport  Port=2
  vtp : Outport  Port=3
  vtp_valid : Outport  Port=4
  hdr : Outport  Port=5
  hdr_valid : Outport  Port=6
  data_out : Outport  Port=7
  data_valid_out : Outport  Port=8
  wires:
  [frame_data] -> diagnose_header_timing/3(frame_pulse)
  [frame_ext] -> diagnose_header_timing/2(hdr_valid)
  [hdr] -> diagnose_header_timing/1(hdr)
  " hdr_w0"/1 -> [w0]
  " hdr_w1"/1 -> [w1]
  " hdr_w2"/1 -> [w2]
  " hdr_w3"/1 -> [w3]
  " hdr_w4"/1 -> [w4]
  " hdr_w5"/1 -> [w5]
  " hdr_w6"/1 -> [w6]
  " hdr_w7"/1 -> [w7]
  sync_in/1 -> sync_out/1
  " data_in"/1 -> data_out/1, [data]
  frame_in/1 -> [frame_pulse], [frame_data], frame_out/1
  Delay/1 -> Mux/3
  Delay1/1 -> Mux/4
  Delay2/1 -> Mux/5
  Delay3/1 -> Mux/6
  Delay4/1 -> Mux/7
  Delay5/1 -> Mux/8
  Delay6/1 -> Mux/9
  Counter/1 -> Mux/1
  [frame_pulse] -> extend_8/1(frame_pulse)
  extend_8/1(frame_pulse_8) -> Counter/1, Mux1/1, [frame_ext]
  [hdr] -> hdr/1
  [frame_ext] -> hdr_valid/1
  [w0] -> Mux/2
  [w1] -> Delay/1
  [w2] -> Delay1/1
  [w3] -> Delay2/1
  [w4] -> Delay3/1
  [w5] -> Delay4/1
  [w6] -> Delay5/1
  [w7] -> Delay6/1
  [data] -> diagnose_header_timing/4(data)
  Mux1/1 -> [hdr]
  Mux/1 -> Mux1/3
  Constant/1 -> Mux1/2
  vtp0/1 -> [vtp0]
  vtp1/1 -> [vtp1]
  [frame_pulse] -> extend_2/1(frame_pulse)
  extend_2/1(frame_pulse_2) -> [vtp_valid], Mux3/1, Counter1/1
  Counter1/1 -> Mux2/1
  Constant1/1 -> Mux3/2
  Mux2/1 -> Mux3/3
  [vtp0] -> Mux2/2
  [vtp1] -> Mux2/3
  Mux3/1 -> [vtp]
  [vtp] -> vtp/1
  [vtp_valid] -> vtp_valid/1
  extend_2048/1(p2048) -> data_valid_out/1
  [frame_pulse] -> extend_2048/1(pulse)

== system uut_vdif/buffer_data/bus_expand ==
  bus_in : Inport
  reinterpret1 : xbsIndex_r4/Reinterpret  force_arith_type=on  arith_type=Unsigned  force_bin_pt=on  bin_pt=0  block_type=reinterpret
  reinterpret2 : xbsIndex_r4/Reinterpret  force_arith_type=on  arith_type=Unsigned  force_bin_pt=on  bin_pt=0  block_type=reinterpret
  slice1 : xbsIndex_r4/Slice  nbits=16  boolean_output=off  mode=Upper Bit Location + Width  bit1=-16  base1=MSB of Input  bit0=0  base0=LSB of Input  dbl_ovrd=off  block_type=slice
  slice2 : xbsIndex_r4/Slice  nbits=16  boolean_output=off  mode=Upper Bit Location + Width  bit1=0  base1=MSB of Input  bit0=0  base0=LSB of Input  dbl_ovrd=off  block_type=slice
  msb_out2 : Outport
  lsb_out1 : Outport  Port=2
  wires:
  reinterpret1/1 -> lsb_out1/1
  slice1/1 -> reinterpret1/1
  reinterpret2/1 -> msb_out2/1
  slice2/1 -> reinterpret2/1
  bus_in/1 -> slice1/1, slice2/1

== system uut_vdif/buffer_data/bus_expand1 ==
  bus_in : Inport
  reinterpret1 : xbsIndex_r4/Reinterpret  force_arith_type=on  arith_type=Unsigned  force_bin_pt=on  bin_pt=0  block_type=reinterpret
  reinterpret2 : xbsIndex_r4/Reinterpret  force_arith_type=on  arith_type=Unsigned  force_bin_pt=on  bin_pt=0  block_type=reinterpret
  slice1 : xbsIndex_r4/Slice  nbits=32  boolean_output=off  mode=Upper Bit Location + Width  bit1=-32  base1=MSB of Input  bit0=0  base0=LSB of Input  dbl_ovrd=off  block_type=slice
  slice2 : xbsIndex_r4/Slice  nbits=32  boolean_output=off  mode=Upper Bit Location + Width  bit1=0  base1=MSB of Input  bit0=0  base0=LSB of Input  dbl_ovrd=off  block_type=slice
  msb_out2 : Outport
  lsb_out1 : Outport  Port=2
  wires:
  reinterpret1/1 -> lsb_out1/1
  slice1/1 -> reinterpret1/1
  reinterpret2/1 -> msb_out2/1
  slice2/1 -> reinterpret2/1
  bus_in/1 -> slice1/1, slice2/1

== system uut_vdif/buffer_data/bus_expand2 ==
  bus_in : Inport
  reinterpret1 : xbsIndex_r4/Reinterpret  force_arith_type=on  arith_type=Unsigned  force_bin_pt=on  bin_pt=0  block_type=reinterpret
  reinterpret2 : xbsIndex_r4/Reinterpret  force_arith_type=on  arith_type=Unsigned  force_bin_pt=on  bin_pt=0  block_type=reinterpret
  slice1 : xbsIndex_r4/Slice  nbits=32  boolean_output=off  mode=Upper Bit Location + Width  bit1=-32  base1=MSB of Input  bit0=0  base0=LSB of Input  dbl_ovrd=off  block_type=slice
  slice2 : xbsIndex_r4/Slice  nbits=32  boolean_output=off  mode=Upper Bit Location + Width  bit1=0  base1=MSB of Input  bit0=0  base0=LSB of Input  dbl_ovrd=off  block_type=slice
  msb_out2 : Outport
  lsb_out1 : Outport  Port=2
  wires:
  bus_in/1 -> slice2/1, slice1/1
  slice2/1 -> reinterpret2/1
  reinterpret2/1 -> msb_out2/1
  slice1/1 -> reinterpret1/1
  reinterpret1/1 -> lsb_out1/1

== system uut_vdif/buffer_data/bus_expand3 ==
  bus_in : Inport
  reinterpret1 : xbsIndex_r4/Reinterpret  force_arith_type=on  arith_type=Unsigned  force_bin_pt=on  bin_pt=0  block_type=reinterpret
  reinterpret2 : xbsIndex_r4/Reinterpret  force_arith_type=on  arith_type=Unsigned  force_bin_pt=on  bin_pt=0  block_type=reinterpret
  slice1 : xbsIndex_r4/Slice  nbits=32  boolean_output=off  mode=Upper Bit Location + Width  bit1=-32  base1=MSB of Input  bit0=0  base0=LSB of Input  dbl_ovrd=off  block_type=slice
  slice2 : xbsIndex_r4/Slice  nbits=32  boolean_output=off  mode=Upper Bit Location + Width  bit1=0  base1=MSB of Input  bit0=0  base0=LSB of Input  dbl_ovrd=off  block_type=slice
  msb_out2 : Outport
  lsb_out1 : Outport  Port=2
  wires:
  reinterpret1/1 -> lsb_out1/1
  slice1/1 -> reinterpret1/1
  reinterpret2/1 -> msb_out2/1
  slice2/1 -> reinterpret2/1
  bus_in/1 -> slice1/1, slice2/1

== system uut_vdif/buffer_data/diagnose_data_valid ==
  data_top : Inport
  data_bott : Inport  Port=2
  valid : Inport  Port=3
  frame_start_out : Inport  Port=4
  Disregard Subsystem : xbsIndex_r4/Disregard Subsystem  Tag=discardX  block_type=disregard
  Gateway Out{1..4} (4 alike) : xbsIndex_r4/Gateway Out  inherit_from_input=off  hdl_port=on  timing_constraint=None  locs_specified=off  LOCs={}  UseAsDAC=off  DACChannel='1'  block_type=gatewayout
  Scope : Scope  NumInputPorts=4
      settings: TimeRange=1.649420126233963  YMin=6.93637e+12~0.95~-1~-5  YMax=7.66651e+12~1.05~1~5
  wires:
  Gateway Out1/1 -> Scope/3  "valid"
  valid/1 -> Gateway Out1/1  "tx_valid"
  data_top/1 -> Gateway Out2/1  "tx_data"
  data_bott/1 -> Gateway Out3/1  "tx_valid"
  Gateway Out2/1 -> Scope/1  "data_top"
  Gateway Out3/1 -> Scope/2  "data_bott"
  Gateway Out4/1 -> Scope/4  "frame_start_out"
  frame_start_out/1 -> Gateway Out4/1  "tx_valid"

== system uut_vdif/buffer_data/diagnose_full ==
  input_data_top : Inport
  input_data_bott : Inport  Port=2
  empty : Inport  Port=3
  full : Inport  Port=4
  pct_full : Inport  Port=5
  we : Inport  Port=6
  Disregard Subsystem : xbsIndex_r4/Disregard Subsystem  Tag=discardX  block_type=disregard
  Gateway Out{1..6} (6 alike) : xbsIndex_r4/Gateway Out  inherit_from_input=off  hdl_port=on  timing_constraint=None  locs_specified=off  LOCs={}  UseAsDAC=off  DACChannel='1'  block_type=gatewayout
  Scope : Scope  NumInputPorts=6
      settings: TimeRange=1.649420126233963  YMin=6.93637e+12~0.95~-1~-5~-5~-5  YMax=7.66651e+12~1.05~1~5~5~5
  wires:
  Gateway Out1/1 -> Scope/3  "empty"
  empty/1 -> Gateway Out1/1  "tx_valid"
  input_data_top/1 -> Gateway Out2/1  "tx_data"
  input_data_bott/1 -> Gateway Out3/1  "tx_valid"
  Gateway Out2/1 -> Scope/1  "input_data_top"
  Gateway Out3/1 -> Scope/2  "input_data_bott"
  Gateway Out4/1 -> Scope/4  "full"
  full/1 -> Gateway Out4/1  "tx_valid"
  Gateway Out5/1 -> Scope/5  "pct_full"
  pct_full/1 -> Gateway Out5/1  "tx_valid"
  Gateway Out6/1 -> Scope/6  "we"
  we/1 -> Gateway Out6/1  "tx_valid"

== system uut_vdif/buffer_data/diagnose_full1 ==
  frame_start : Inport
  empty : Inport  Port=2
  full : Inport  Port=3
  pct_full : Inport  Port=4
  we : Inport  Port=5
  Disregard Subsystem : xbsIndex_r4/Disregard Subsystem  Tag=discardX  block_type=disregard
  Gateway Out{1..2,4..6} (5 alike) : xbsIndex_r4/Gateway Out  inherit_from_input=off  hdl_port=on  timing_constraint=None  locs_specified=off  LOCs={}  UseAsDAC=off  DACChannel='1'  block_type=gatewayout
  Scope : Scope  NumInputPorts=5
      settings: TimeRange=1.649420126233963  YMin=-1~-1~0.984375~1~1  YMax=1~1~0.984375~1~1
  wires:
  we/1 -> Gateway Out6/1  "tx_valid"
  pct_full/1 -> Gateway Out5/1  "tx_valid"
  full/1 -> Gateway Out4/1  "tx_valid"
  Gateway Out2/1 -> Scope/1  "frame_start"
  frame_start/1 -> Gateway Out2/1  "tx_data"
  empty/1 -> Gateway Out1/1  "tx_valid"
  Gateway Out1/1 -> Scope/2  "empty"
  Gateway Out4/1 -> Scope/3  "full"
  Gateway Out6/1 -> Scope/5  "we"
  Gateway Out5/1 -> Scope/4  "pct_full"

== system uut_vdif/buffer_data/diagnose_hdr_valid ==
  hdr_top : Inport
  hdr_bott : Inport  Port=2
  valid : Inport  Port=3
  sync_out : Inport  Port=4
  Disregard Subsystem : xbsIndex_r4/Disregard Subsystem  Tag=discardX  block_type=disregard
  Gateway Out{1..4} (4 alike) : xbsIndex_r4/Gateway Out  inherit_from_input=off  hdl_port=on  timing_constraint=None  locs_specified=off  LOCs={}  UseAsDAC=off  DACChannel='1'  block_type=gatewayout
  Scope : Scope  NumInputPorts=4
      settings: TimeRange=1.649420126233963  YMin=6.93637e+12~0.95~-1~-5  YMax=7.66651e+12~1.05~1~5
  wires:
  sync_out/1 -> Gateway Out4/1  "tx_valid"
  Gateway Out4/1 -> Scope/4  "sync_out"
  Gateway Out3/1 -> Scope/2  "hdr_bott"
  Gateway Out2/1 -> Scope/1  "hdr_top"
  hdr_bott/1 -> Gateway Out3/1  "tx_valid"
  hdr_top/1 -> Gateway Out2/1  "tx_data"
  valid/1 -> Gateway Out1/1  "tx_valid"
  Gateway Out1/1 -> Scope/3  "valid"

== system uut_vdif/buffer_data/diagnose_input_data ==
  input_data_top : Inport
  input_data_bott : Inport  Port=2
  valid : Inport  Port=3
  frame_start_int : Inport  Port=4
  Disregard Subsystem : xbsIndex_r4/Disregard Subsystem  Tag=discardX  block_type=disregard
  Gateway Out{1..4} (4 alike) : xbsIndex_r4/Gateway Out  inherit_from_input=off  hdl_port=on  timing_constraint=None  locs_specified=off  LOCs={}  UseAsDAC=off  DACChannel='1'  block_type=gatewayout
  Scope : Scope  NumInputPorts=4
      settings: TimeRange=1.649420126233963  YMin=6.93637e+12~0.95~-1~-5  YMax=7.66651e+12~1.05~1~5
  wires:
  frame_start_int/1 -> Gateway Out4/1  "tx_valid"
  Gateway Out4/1 -> Scope/4  "frame_start_out"
  Gateway Out3/1 -> Scope/2  "input_data_bott"
  Gateway Out2/1 -> Scope/1  "input_data_top"
  input_data_bott/1 -> Gateway Out3/1  "tx_valid"
  input_data_top/1 -> Gateway Out2/1  "tx_data"
  valid/1 -> Gateway Out1/1  "tx_valid"
  Gateway Out1/1 -> Scope/3  "valid"

== system uut_vdif/buffer_data/extend_1024 ==
  pulse : Inport
  Delay1 : xbsIndex_r4/Delay  rst=off  infoeditControl=Selection of Reset will increase slice count due to use of real FFs and instead of SRLs  en=off  latency=1  dbl_ovrd=off  reg_retiming=off  block_type=delay
  Delay10 : xbsIndex_r4/Delay  rst=off  infoeditControl=Selection of Reset will increase slice count due to use of real FFs and instead of SRLs  en=off  latency=512  dbl_ovrd=off  reg_retiming=off  block_type=delay
  Delay2 : xbsIndex_r4/Delay  rst=off  infoeditControl=Selection of Reset will increase slice count due to use of real FFs and instead of SRLs  en=off  latency=2  dbl_ovrd=off  reg_retiming=off  block_type=delay
  Delay3 : xbsIndex_r4/Delay  rst=off  infoeditControl=Selection of Reset will increase slice count due to use of real FFs and instead of SRLs  en=off  latency=4  dbl_ovrd=off  reg_retiming=off  block_type=delay
  Delay4 : xbsIndex_r4/Delay  rst=off  infoeditControl=Selection of Reset will increase slice count due to use of real FFs and instead of SRLs  en=off  latency=8  dbl_ovrd=off  reg_retiming=off  block_type=delay
  Delay5 : xbsIndex_r4/Delay  rst=off  infoeditControl=Selection of Reset will increase slice count due to use of real FFs and instead of SRLs  en=off  latency=16  dbl_ovrd=off  reg_retiming=off  block_type=delay
  Delay6 : xbsIndex_r4/Delay  rst=off  infoeditControl=Selection of Reset will increase slice count due to use of real FFs and instead of SRLs  en=off  latency=32  dbl_ovrd=off  reg_retiming=off  block_type=delay
  Delay7 : xbsIndex_r4/Delay  rst=off  infoeditControl=Selection of Reset will increase slice count due to use of real FFs and instead of SRLs  en=off  latency=64  dbl_ovrd=off  reg_retiming=off  block_type=delay
  Delay8 : xbsIndex_r4/Delay  rst=off  infoeditControl=Selection of Reset will increase slice count due to use of real FFs and instead of SRLs  en=off  latency=128  dbl_ovrd=off  reg_retiming=off  block_type=delay
  Delay9 : xbsIndex_r4/Delay  rst=off  infoeditControl=Selection of Reset will increase slice count due to use of real FFs and instead of SRLs  en=off  latency=256  dbl_ovrd=off  reg_retiming=off  block_type=delay
  Logical{1..10} (10 alike) : xbsIndex_r4/Logical  logical_function=OR  inputs=2  en=off  latency=0  precision=Full  arith_type=Unsigned  n_bits=16  bin_pt=0  align_bp=on  dbl_ovrd=off  block_type=logical
  p1024 : Outport
  wires:
  Delay2/1 -> Logical2/2
  Logical1/1 -> Logical2/1, Delay2/1
  Delay1/1 -> Logical1/2
  pulse/1 -> Logical1/1, Delay1/1
  Logical2/1 -> Delay3/1, Logical3/1
  Delay3/1 -> Logical3/2
  Logical3/1 -> Delay4/1, Logical4/1
  Delay4/1 -> Logical4/2
  Logical4/1 -> Logical5/1, Delay5/1
  Delay5/1 -> Logical5/2
  Logical5/1 -> Delay6/1, Logical6/1
  Delay6/1 -> Logical6/2
  Logical6/1 -> Logical7/1, Delay7/1
  Delay7/1 -> Logical7/2
  Logical7/1 -> Delay8/1, Logical8/1
  Delay8/1 -> Logical8/2
  Logical8/1 -> Logical9/1, Delay9/1
  Delay9/1 -> Logical9/2
  Logical9/1 -> Delay10/1, Logical10/1
  Delay10/1 -> Logical10/2
  Logical10/1 -> p1024/1

== system uut_vdif/buffer_data/extend_4 ==
  pulse : Inport
  Delay1 : xbsIndex_r4/Delay  rst=off  infoeditControl=Selection of Reset will increase slice count due to use of real FFs and instead of SRLs  en=off  latency=1  dbl_ovrd=off  reg_retiming=off  block_type=delay
  Delay2 : xbsIndex_r4/Delay  rst=off  infoeditControl=Selection of Reset will increase slice count due to use of real FFs and instead of SRLs  en=off  latency=2  dbl_ovrd=off  reg_retiming=off  block_type=delay
  Logical1 : xbsIndex_r4/Logical  logical_function=OR  inputs=2  en=off  latency=0  precision=Full  arith_type=Unsigned  n_bits=16  bin_pt=0  align_bp=on  dbl_ovrd=off  block_type=logical
  Logical2 : xbsIndex_r4/Logical  logical_function=OR  inputs=2  en=off  latency=0  precision=Full  arith_type=Unsigned  n_bits=16  bin_pt=0  align_bp=on  dbl_ovrd=off  block_type=logical
  pulse_4 : Outport
  wires:
  pulse/1 -> Delay1/1, Logical1/1
  Logical2/1 -> pulse_4/1
  Delay1/1 -> Logical1/2
  Logical1/1 -> Delay2/1, Logical2/1
  Delay2/1 -> Logical2/2

== system uut_vdif/buffer_data/rst ==
  sim_1 : Inport
  io_delay : xbsIndex_r4/Delay  rst=off  infoeditControl=Selection of Reset will increase slice count due to use of real FFs and instead of SRLs  en=off  latency=0  dbl_ovrd=off  reg_retiming=on  block_type=delay
  reint1 : xbsIndex_r4/Reinterpret  force_arith_type=on  arith_type=Unsigned  force_bin_pt=on  bin_pt=0  block_type=reinterpret
  slice_reg : xbsIndex_r4/Slice  nbits=32  boolean_output=off  mode=Lower Bit Location + Width  bit1=0  base1=MSB of Input  bit0=0  base0=LSB of Input  dbl_ovrd=off  block_type=slice
  uut_vdif_buffer_data_rst_user_data_out : xbsIndex_r4/Gateway In  gui_display_data_type=Fixed-point  arith_type=Unsigned  n_bits=32  bin_pt=0  preci_type=Single  exp_width=8  frac_width=24  quantization="Round  (unbiased: +/- Inf)"  overflow=Saturate  period=1  dbl_ovrd=off  timing_constraint=None  locs_specified=off  LOCs={}  UseAsADC=off  ADCChannel='1'  inherit_from_input=off  hdl_port=on  block_type=gatewayin
  in_reg : Outport
  wires:
  uut_vdif_buffer_data_rst_user_data_out/1 -> io_delay/1
  sim_1/1 -> uut_vdif_buffer_data_rst_user_data_out/1
  io_delay/1 -> slice_reg/1
  slice_reg/1 -> reint1/1
  reint1/1 -> in_reg/1
